simulink model "fun_ut"  (Simulink 7.0)
settings: Solver=FixedStepDiscrete  StartTime=0.0  StopTime=10.0  FixedStep=C_TICK_TIME_S  RelTol=1e-3
PreLoadFcn:
  | if exist('tl_preloadfcn','file'), tl_preloadfcn(gcs,100); end
PostLoadFcn:
  | if exist('tl_postloadfcn','file'), tl_postloadfcn(gcs,100); end
InitFcn:
  | if exist('tlds_init','file'), tlds_init(gcs); end
StartFcn:
  | if exist('tlds_start','file'), tlds_start(gcs); end
StopFcn:
  | if exist('tlds_stop','file'), tlds_stop(gcs); end
undefined symbols (not defined in the file or in its folder): VINP_HVBattPwrAvailDischargeValid_flg, VINP_HVBattSOC_pct, VINP_HVBattSOCValid_flg, VINP_MCUEnabled_flg
libraries: siltestlib x5, fun x1, simulink x1
PreSaveFcn:
  | if exist('tl_presavefcn','file'), tl_presavefcn(gcs); end
settings Model: DS_PROJECTFILE=hcu_strategy.dd  TL_MAIN_DATA=struct('date',733922.63123271987,'maxnumsimulations',10,'codeopt',struct('inliningthreshold',6,'target',['Generic ANSI-C'],'assembler',0,'optlevel',2,'linebreaklimit',100,'stateactcodinglimit',5,'functionsfor64bitops',1,'sections',1,'sfbitfields',1,'globalbitfields',0,'sharefunctions',0,'noinitstozero',0,'limidentlength',1,'decimals',1,'separatesearch',0,'cleancode',0,'optimizedbooltype',1,'keepsaturation',0,'extvarsharing',0,'outputstylefile','cconfig.xml','rootstylesheet','TL_CSourceCodeSS.xsl','addchecksum',0,'modelsaving',2,'browsecodegen',0),'frameopt',struct('exectime',1,'stacksize',1,'simconfig',['default EVM'],'targettimeout',1,'mexargs','-g','tcargs',''),'logopt',struct('plotinterval',inf,'globalloggingmode',1),'export',struct('directory','.\export','sysfiles',1,'docfiles',0,'tools',0),'codecoveragelevel',0,'asapscript','asap2_all_in_one','docscript','tldoc_default','rtos',struct('enablemultirate',0,'currentrtos',['generic RTOS'],'autopriority',0,'autoinitalarm',1,'alarminitwithrestart',1,'usestartuphook',0,'useshutdownhook',0,'usepretaskhook',0,'useposttaskhook',0,'useerrorhook',0,'alarmactivationkind',1,'alarmstartoffset',0),'blockcomment','')  TLRevision=100  Creator=pg2  LastModifiedBy=eb8  BufferReuse=off
settings DataIOCC: LimitDataPoints=off  SaveOutput=off  SaveTime=off
settings OptimizationCC: BlockReduction=off  OptimizeBlockIOStorage=off  BufferReuse=off  ExpressionFolding=off  LocalBlockOutputs=off
settings DebuggingCC: SignalInfNanChecking=warning  SaveWithParameterizedLinksMsg=none  SignalResolutionControl=TryResolveAllWithWarning  InheritedTsInSrcMsg=none  UniqueDataStoreMsg=warning
settings GRTTargetCC: TargetFcnLib=ansi_tfl_tmw.mat

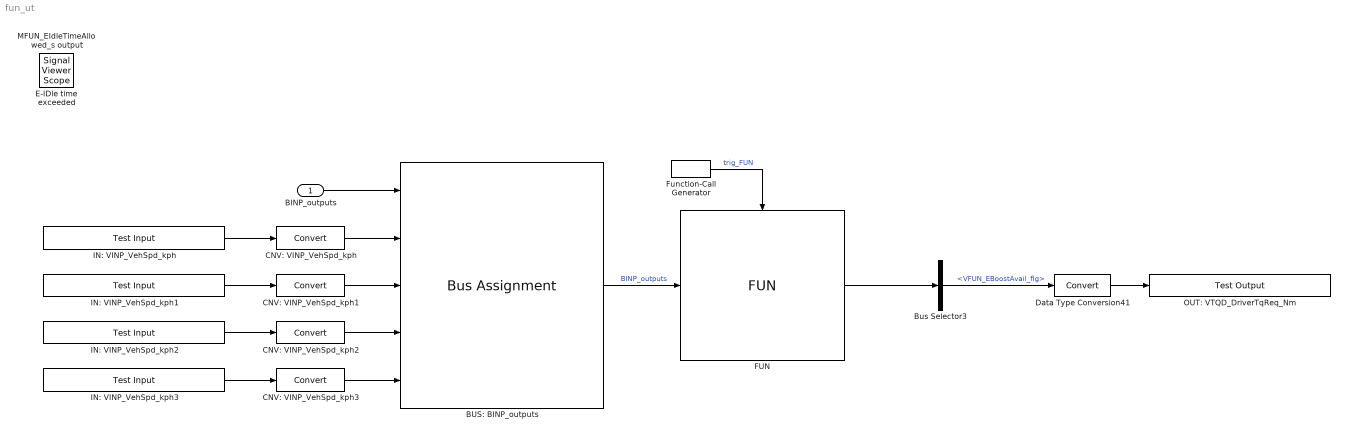
== system fun_ut ==
  BINP_outputs : Inport  UseBusObject=on  OutDataType=fixdt(1, 16)  OutScaling=2^0
      settings: BusObject=BINP_outputs
  BUS: BINP_outputs : BusAssignment  AssignedSignals=VINP_HVBattSOC_pct,VINP_HVBattSOCValid_flg,VINP_HVBattPwrAvailDischargeValid_flg,VINP_MCUEnabled_flg
  Bus Selector3 : BusSelector  OutputSignals=VFUN_EBoostAvail_flg
  CNV: VINP_VehSpd_kph : DataTypeConversion  OutDataTypeMode=double  OutDataType=fixdt(1, 16)  OutScaling=2^0
  CNV: VINP_VehSpd_kph1 : DataTypeConversion  OutDataTypeMode=boolean  OutDataType=fixdt(1, 16)  OutScaling=2^0
  CNV: VINP_VehSpd_kph2 : DataTypeConversion  OutDataTypeMode=boolean  OutDataType=fixdt(1, 16)  OutScaling=2^0
  CNV: VINP_VehSpd_kph3 : DataTypeConversion  OutDataTypeMode=boolean  OutDataType=fixdt(1, 16)  OutScaling=2^0
  Data Type Conversion41 : DataTypeConversion  OutDataType=fixdt(1, 16)  OutScaling=2^0
  FUN : fun/FUN  SystemSampleTime=-1
  Function-Call Generator : simulink/Ports & Subsystems/Function-Call Generator  sample_time=C_TICK_TIME_S  numberOfIterations=1
  IN: VINP_VehSpd_kph : siltestlib/Test Input  varname=VINP_HVBattSOC_pct  sampletime=-1
  IN: VINP_VehSpd_kph1 : siltestlib/Test Input  varname=VINP_HVBattSOCValid_flg  sampletime=-1
  IN: VINP_VehSpd_kph2 : siltestlib/Test Input  varname=VINP_HVBattPwrAvailDischargeValid_flg  sampletime=-1
  IN: VINP_VehSpd_kph3 : siltestlib/Test Input  varname=VINP_MCUEnabled_flg  sampletime=-1
  OUT: VTQD_DriverTqReq_Nm : siltestlib/Test Output  varname=VFUN_EBoostAvail_flg  sampletime=-1
  E-IDle time exceeded : SignalViewerScope  IOType=viewer  RefreshTime=0.035000
  MFUN_EIdleTimeAllowed_s output : SignalViewerScope  IOType=viewer  RefreshTime=0.035000
  wires:
  Function-Call Generator/1 -> FUN/Trigger  "trig_FUN"
  BUS: BINP_outputs/1 -> FUN/1  "BINP_outputs"
  FUN/1 -> Bus Selector3/1
  IN: VINP_VehSpd_kph/1 -> CNV: VINP_VehSpd_kph/1
  BINP_outputs/1 -> BUS: BINP_outputs/1
  CNV: VINP_VehSpd_kph/1 -> BUS: BINP_outputs/2
  IN: VINP_VehSpd_kph1/1 -> CNV: VINP_VehSpd_kph1/1
  IN: VINP_VehSpd_kph2/1 -> CNV: VINP_VehSpd_kph2/1
  IN: VINP_VehSpd_kph3/1 -> CNV: VINP_VehSpd_kph3/1
  CNV: VINP_VehSpd_kph1/1 -> BUS: BINP_outputs/3
  CNV: VINP_VehSpd_kph2/1 -> BUS: BINP_outputs/4
  CNV: VINP_VehSpd_kph3/1 -> BUS: BINP_outputs/5
  Data Type Conversion41/1 -> OUT: VTQD_DriverTqReq_Nm/1
  Bus Selector3/1 -> Data Type Conversion41/1  "<VFUN_EBoostAvail_flg>"
